simulink model "sampleModel1563"  (R2023a)
settings: Solver=VariableStepAuto  StartTime=0.0  StopTime=10.0  RelTol=1e-3
libraries: hdlsllib x4
settings Model: Creator=user1  LastModifiedBy=user1

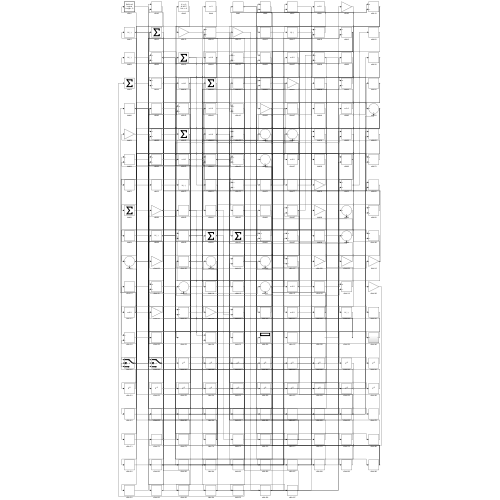
[thumbnail: Simulink's stored preview of the top-level diagram]
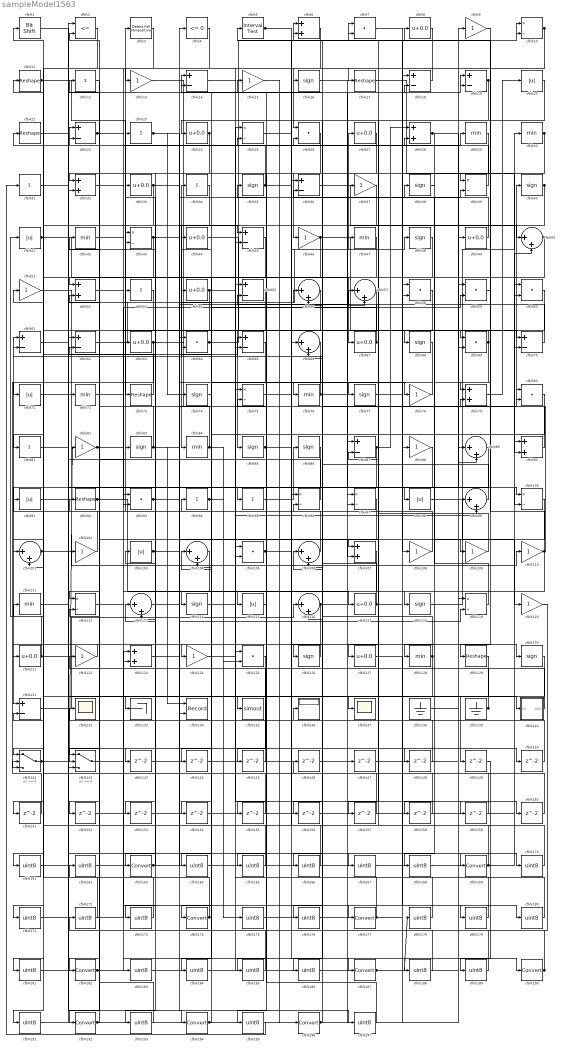
== system sampleModel1563 ==
  cfblk1 : hdlsllib/Logic and Bit Operations/Bit Shift  mode=Shift Left Logical  N=0
  cfblk{10,25,39,43,75,96..97,100,112,119} (10 alike) : Product  Inputs=*/  RndMeth=Zero  SaturateOnIntegerOverflow=on
  cfblk{50,56..57,66,89,99,101,104,106,113,116} (11 alike) : Sum  Inputs=|++
  cfblk{9,13,15,37,46,51,78,82,88,102,108..110,120,122,124} (16 alike) : Gain
  cfblk{20,41,71,91,98,103,115} (7 alike) : Abs  SaturateOnIntegerOverflow=off
  cfblk{7,26,58..60,64,69,80,93,105,125} (11 alike) : DotProduct  OutDataTypeStr=Inherit: Inherit via internal rule
  cfblk{6,28,32,52,79,90,107,123} (8 alike) : Sum
  cfblk{11,17,21,73,92,129} (6 alike) : Reshape
  cfblk{29..30,42,47,72,76,84,111,128} (9 alike) : MinMax
  cfblk{16,35,38,40,48,68,74,77,83,85..86,114,118,126,130} (15 alike) : Signum
  cfblk{8,24,27,33,44,49,54,63,67,117,121,127} (12 alike) : Bias  Bias=0.0  SaturateOnIntegerOverflow=off
  cfblk{12,23,31,34,53,81,94..95} (8 alike) : Sum  Inputs=+
  cfblk{14,18..19,22,36,45,55,61..62,65,70,87,131} (13 alike) : Sum  Inputs=+-
  cfblk132 : Scope
  cfblk133 : Terminator
  cfblk134 : Record  FileSettingsInternal="{\"entries\":[{\"content\":{\"excelSettings\":{\"content\":{},\"type\":\"Streamout.ExcelSettings\"}},\"type\":\"Streamout.FileSettingStorage\",\"uuid\":\"\"}],\"packageUris\":[\"http:\\/\\/schema.mathworks.com\\/mf0\\/streamout_blocks\\/R2020a\"],\"version\":\"1.0\"}"  Layout=[1 1]  SignalsInternal="{\"entries\":[{\"content\":{\"signals\":[{\"content\":{\"blockPath\":[],\"dimensions\":[1],\"domain\":\"\",\"lineColor\":\"#a2142f\",\"plots\":[1],\"port\":1,\"signalID\":1710,\"signalName\":\"XY Graph:1\"},\"type\":\"RecordBlkView.Signal\",\"uuid\":\"\"},{\"content\":{\"blockPath\":[],\"dimensions\":[1],\"domain\":\"\",\"lineColor\":\"#139fff\",\"plots\":[1],\"port\":2,\"signalID\":1713,\"signalName\":\"XY Graph:2\"},\"type\":\"RecordBlkView.Signal\",\"uuid\":\"\"}]},\"type\":\"RecordBlkView.InputSignals\",\"uuid\":\"\"}],\"packageUris\":[\"http:\\/\\/schema.mathworks.com\\/mf0\\/streamout_blocks\\/R2020a\"],\"version\":\"1.0\"}"  VisualizationBindings="{\"xyplotplugin\":{\"info\":[{\"series\":[{\"bindingParametersList\":[{\"parameter\":\"X-Axis\",\"signalID\":1710,\"signalName\":\"XY Graph:1\"},{\"parameter\":\"Y-Axis\",\"signalID\":1713,\"signalName\":\"XY Graph:2\"}],\"seriesID\":28745}],\"subplotID\":1}]}}"  CompatibilityTag=XY  st=-1
  cfblk135 : ToWorkspace  VariableName=simout  SaveFormat=Timeseries  SampleTime=-1
  cfblk136 : Display
  cfblk137 : Scope
  cfblk138 : Ground
  cfblk139 : Ground
  cfblk140 : Subsystem
      settings: LibrarySourceBlock=|
      | hdlsllib/Ports &
      | Subsystems/Subsystem
  cfblk141 : Switch  SaturateOnIntegerOverflow=off  InputSameDT=off
  cfblk142 : Switch  SaturateOnIntegerOverflow=off  InputSameDT=off
  cfblk{143..160} (18 alike) : Delay  SampleTime=1
  cfblk{161..162,164..168,170..173,175..176,178..181,183..186,188..189,191,193,195,197} (27 alike) : DataTypeConversion  OutDataTypeStr=uint8  SaturateOnIntegerOverflow=off  RndMeth=Floor
  cfblk{163,169,174,177,182,187,190,192,194,196} (10 alike) : DataTypeConversion  SaturateOnIntegerOverflow=off  RndMeth=Floor
  cfblk2 : RelationalOperator  Operator=<=  OutDataTypeStr=boolean  InputSameDT=off
  cfblk3 : hdlsllib/Logic and Bit Operations/Detect Fall Nonpositive  vinit=0  OutDataTypeStr=boolean
  cfblk4 : hdlsllib/Logic and Bit Operations/Compare To Zero  relop=<=  OutDataTypeStr=boolean
  cfblk5 : hdlsllib/Logic and Bit Operations/Interval Test  IntervalClosedRight=on  uplimit=0.5  IntervalClosedLeft=on  lowlimit=-0.5  OutDataTypeStr=boolean
  wires:
  cfblk106/1 -> cfblk3/1
  cfblk8/1 -> cfblk17/1
  cfblk79/1 -> cfblk20/1
  cfblk69/1 -> cfblk68/1, cfblk168/1
  cfblk30/1 -> cfblk193/1, cfblk195/1
  cfblk18/1 -> cfblk13/1
  cfblk131/1 -> cfblk116/1
  cfblk51/1 -> cfblk110/1
  cfblk108/1 -> cfblk61/1
  cfblk63/1 -> cfblk40/1, cfblk141/3
  cfblk126/1 -> cfblk124/1
  cfblk121/1 -> cfblk41/1, cfblk18/2
  cfblk138/1 -> cfblk9/1
  cfblk89/1 -> cfblk131/1
  cfblk26/1 -> cfblk32/1
  cfblk141/1 -> cfblk82/1, cfblk56/1
  cfblk7/1 -> cfblk108/1
  cfblk33/1 -> cfblk142/1, cfblk140/1(In1)
  cfblk21/1 -> cfblk32/2
  cfblk95/1 -> cfblk86/1
  cfblk78/1 -> cfblk76/1
  cfblk118/1 -> cfblk30/1
  cfblk64/1 -> cfblk8/1, cfblk160/1
  cfblk43/1 -> cfblk52/1, cfblk77/1
  cfblk16/1 -> cfblk98/1
  cfblk29/1 -> cfblk73/1
  cfblk73/1 -> cfblk21/1
  cfblk13/1 -> cfblk78/1
  cfblk27/1 -> cfblk46/1
  cfblk31/1 -> cfblk194/1
  cfblk41/1 -> cfblk67/1, cfblk134/2, cfblk135/1
  cfblk54/1 -> cfblk101/1, cfblk99/2
  cfblk87/1 -> cfblk28/1, cfblk191/1
  cfblk9/1 -> cfblk79/1
  cfblk44/1 -> cfblk69/1
  cfblk40/1 -> cfblk84/1, cfblk127/1
  cfblk75/1 -> cfblk177/1
  cfblk28/1 -> cfblk118/1, cfblk100/2
  cfblk48/1 -> cfblk133/1
  cfblk42/1 -> cfblk93/1
  cfblk128/1 -> cfblk61/2, cfblk5/1, cfblk176/1
  cfblk35/1 -> cfblk1/1, cfblk10/2
  cfblk76/1 -> cfblk34/1, cfblk19/1
  cfblk85/1 -> cfblk115/1, cfblk48/1
  cfblk109/1 -> cfblk7/1
  cfblk111/1 -> cfblk169/1
  cfblk10/1 -> cfblk26/1, cfblk39/1, cfblk16/1
  cfblk12/1 -> cfblk192/1
  cfblk119/1 -> cfblk38/1
  cfblk55/1 -> cfblk85/1
  cfblk102/1 -> cfblk11/1
  cfblk84/1 -> cfblk22/1, cfblk175/1
  cfblk100/1 -> cfblk128/1
  cfblk37/1 -> cfblk126/1
  cfblk114/1 -> cfblk55/1
  cfblk46/1 -> cfblk89/2, cfblk91/1
  cfblk103/1 -> cfblk109/1, cfblk39/2
  cfblk17/1 -> cfblk90/2
  cfblk34/1 -> cfblk141/1
  cfblk1/1 -> cfblk102/1
  cfblk92/1 -> cfblk117/1, cfblk59/2, cfblk179/1
  cfblk11/1 -> cfblk53/1, cfblk95/1
  cfblk93/1 -> cfblk79/2, cfblk57/1
  cfblk104/1 -> cfblk163/1
  cfblk110/1 -> cfblk6/1, cfblk80/2, cfblk123/2
  cfblk36/1 -> cfblk50/1
  cfblk96/1 -> cfblk62/2
  cfblk97/1 -> cfblk182/1
  cfblk15/1 -> cfblk196/1
  cfblk83/1 -> cfblk33/1, cfblk37/1, cfblk134/1, cfblk22/2
  cfblk14/1 -> cfblk100/1
  cfblk39/1 -> cfblk23/1
  cfblk71/1 -> cfblk43/1
  cfblk105/1 -> cfblk130/1, cfblk148/1
  cfblk70/1 -> cfblk55/2
  cfblk59/1 -> cfblk129/1
  cfblk50/1 -> cfblk142/2, cfblk106/2, cfblk65/2, cfblk186/1
  cfblk99/1 -> cfblk6/2
  cfblk24/1 -> cfblk152/1, cfblk153/1
  cfblk25/1 -> cfblk187/1
  cfblk67/1 -> cfblk35/1, cfblk14/2
  cfblk53/1 -> cfblk71/1
  cfblk49/1 -> cfblk26/2
  cfblk139/1 -> cfblk122/1, cfblk112/2
  cfblk77/1 -> cfblk10/1
  cfblk101/1 -> cfblk83/1, cfblk19/2
  cfblk122/1 -> cfblk121/1
  cfblk124/1 -> cfblk29/1
  cfblk107/1 -> cfblk113/2
  cfblk98/1 -> cfblk120/1
  cfblk3/1 -> cfblk93/2
  cfblk117/1 -> cfblk14/1, cfblk80/1
  cfblk123/1 -> cfblk119/2
  cfblk57/1 -> cfblk81/1
  cfblk82/1 -> cfblk137/1, cfblk112/1
  cfblk22/1 -> cfblk70/1, cfblk28/2
  cfblk90/1 -> cfblk36/2
  cfblk62/1 -> cfblk27/1
  cfblk20/1 -> cfblk24/1
  cfblk5/1 -> cfblk70/2, cfblk107/2
  cfblk72/1 -> cfblk190/1
  cfblk23/1 -> cfblk45/1, cfblk74/1
  cfblk58/1 -> cfblk174/1
  cfblk88/1 -> cfblk114/1
  cfblk116/1 -> cfblk87/1, cfblk142/3
  cfblk6/1 -> cfblk45/2
  cfblk19/1 -> cfblk107/1, cfblk56/2, cfblk156/1
  cfblk81/1 -> cfblk65/1
  cfblk94/1 -> cfblk44/1, cfblk125/2
  cfblk140/1(Out1) -> cfblk63/1
  cfblk61/1 -> cfblk143/1
  cfblk143/1 -> cfblk89/1
  cfblk45/1 -> cfblk144/1
  cfblk144/1 -> cfblk66/1
  cfblk125/1 -> cfblk145/1
  cfblk145/1 -> cfblk43/2
  cfblk146/1 -> cfblk96/2
  cfblk148/1 -> cfblk87/2
  cfblk129/1 -> cfblk149/1
  cfblk112/1 -> cfblk150/1
  cfblk150/1 -> cfblk62/1
  cfblk56/1 -> cfblk151/1
  cfblk151/1 -> cfblk141/2
  cfblk152/1 -> cfblk36/1
  cfblk153/1 -> cfblk64/1
  cfblk65/1 -> cfblk154/1
  cfblk154/1 -> cfblk90/1
  cfblk115/1 -> cfblk155/1
  cfblk155/1 -> cfblk113/1
  cfblk156/1 -> cfblk50/2
  cfblk68/1 -> cfblk157/1
  cfblk157/1 -> cfblk52/2
  cfblk38/1 -> cfblk158/1
  cfblk158/1 -> cfblk101/2
  cfblk127/1 -> cfblk159/1
  cfblk159/1 -> cfblk116/2
  cfblk160/1 -> cfblk131/2
  cfblk4/1 -> cfblk161/1
  cfblk161/1 -> cfblk49/1
  cfblk162/1 -> cfblk4/1
  cfblk163/1 -> cfblk99/1, cfblk103/1
  cfblk80/1 -> cfblk164/1
  cfblk164/1 -> cfblk104/1
  cfblk66/1 -> cfblk165/1
  cfblk165/1 -> cfblk104/2
  cfblk60/1 -> cfblk166/1
  cfblk166/1 -> cfblk92/1
  cfblk91/1 -> cfblk167/1
  cfblk167/1 -> cfblk60/1
  cfblk168/1 -> cfblk60/2
  cfblk169/1 -> cfblk7/2, cfblk96/1
  cfblk52/1 -> cfblk170/1
  cfblk170/1 -> cfblk111/1
  cfblk2/1 -> cfblk171/1
  cfblk171/1 -> cfblk123/1
  cfblk120/1 -> cfblk172/1
  cfblk172/1 -> cfblk2/1
  cfblk86/1 -> cfblk173/1
  cfblk173/1 -> cfblk2/2
  cfblk174/1 -> cfblk51/1, cfblk42/1
  cfblk175/1 -> cfblk58/1
  cfblk176/1 -> cfblk58/2
  cfblk177/1 -> cfblk146/1, cfblk125/1
  cfblk178/1 -> cfblk75/1
  cfblk179/1 -> cfblk75/2
  cfblk147/1 -> cfblk180/1
  cfblk180/1 -> cfblk105/1
  cfblk130/1 -> cfblk181/1
  cfblk181/1 -> cfblk147/1
  cfblk182/1 -> cfblk178/1, cfblk105/2
  cfblk32/1 -> cfblk183/1
  cfblk183/1 -> cfblk97/1
  cfblk74/1 -> cfblk184/1
  cfblk184/1 -> cfblk97/2
  cfblk47/1 -> cfblk185/1
  cfblk185/1 -> cfblk54/1
  cfblk186/1 -> cfblk47/1
  cfblk187/1 -> cfblk18/1, cfblk59/1
  cfblk142/1 -> cfblk188/1
  cfblk188/1 -> cfblk25/1
  cfblk149/1 -> cfblk189/1
  cfblk189/1 -> cfblk25/2
  cfblk190/1 -> cfblk64/2, cfblk132/1, cfblk66/2, cfblk136/1
  cfblk191/1 -> cfblk72/1
  cfblk192/1 -> cfblk162/1, cfblk119/1
  cfblk193/1 -> cfblk12/1
  cfblk194/1 -> cfblk69/2, cfblk94/1
  cfblk195/1 -> cfblk31/1
  cfblk196/1 -> cfblk57/2, cfblk88/1, cfblk106/1
  cfblk113/1 -> cfblk197/1
  cfblk197/1 -> cfblk15/1

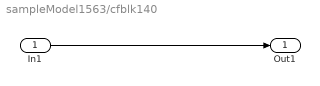
== system sampleModel1563/cfblk140 ==
  In1 : Inport
  Out1 : Outport
  wires:
  In1/1 -> Out1/1
